simulink model "tigor_ev"  (R2020a)
settings: Solver=FixedStepDiscrete  StartTime=0.0  StopTime=0.4  RelTol=1e-3
InitFcn:
  | NAvg = 100;
  | Fs = 1e6;
  | FrameSize = 64;
libraries: dspsrcs4 x2, dspmisc x1
CloseFcn:
  | clear NAvg FrameSize Fs
settings Model: SnapshotInterval=1  Creator=The MathWorks, Inc.  LastModifiedBy=sateeshk
settings DataIOCC: LimitDataPoints=on  SaveFormat=Array  SaveOutput=off  SignalLogging=off  DSMLogging=off  SaveTime=off  ReturnWorkspaceOutputs=off
settings OptimizationCC: LifeSpan=inf
settings DebuggingCC: SolverPrmCheckMsg=warning  AllowSymbolicDim=off  SFUnexpectedBacktrackingDiag=warning  SFNoUnconditionalDefaultTransitionDiag=warning  SFExecutionAtInitializationDiag=none  ArithmeticOperatorsInVariantConditions=warning
settings HardwareCC: ProdBitPerPointer=32  ProdBitPerSizeT=32  ProdBitPerPtrDiffT=32  ProdLargestAtomicFloat=None  ProdIntDivRoundTo=Undefined  ProdEndianess=Unspecified  ProdWordSize=32  ProdHWDeviceType=32-bit Generic
settings ModelReferenceCC: PropagateSignalLabelsOutOfModel=off
settings SFSimCC: SimUseLocalCustomCode=off  CustomCodeUndefinedFunction=UseInterfaceOnly
settings RTWCC: RTWUseLocalCustomCode=off
settings CodeAppCC: StateflowObjectComments=on
settings GRTTargetCC: TargetLangStandard=C89/C90 (ANSI)
settings ConfigComp: CovMetricSettings=dw  CovHtmlReporting=on  CovSaveCumulativeToWorkspaceVar=on  CovSaveSingleToWorkspaceVar=on  CovExternalEMLEnable=off  CovSFcnEnable=off

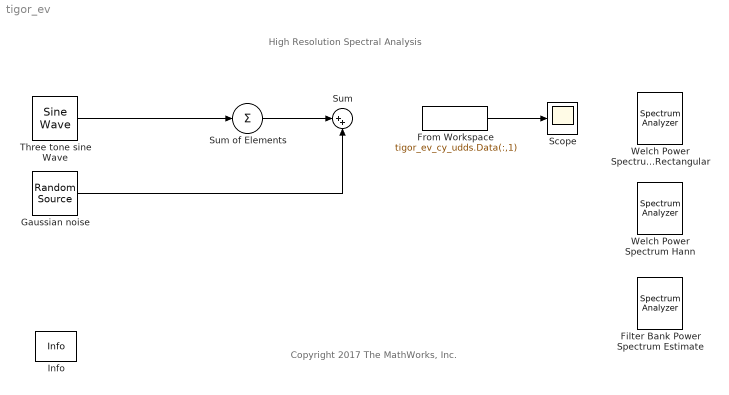
== system tigor_ev ==
  note: High Resolution Spectral Analysis
  note: Copyright 2017 The MathWorks, Inc.
  Filter Bank Power Spectrum Estimate : SpectrumAnalyzer
  From Workspace : FromWorkspace  VariableName=tigor_ev_cy_udds.Data(:,1)  SampleTime=-1
  Gaussian noise : dspsrcs4/Random Source  SrcType=Gaussian  NormMethod=Ziggurat  CltLength=12  MinVal=0  MaxVal=1  MeanVal=0  VarVal=1e-11  RepMode=Specify seed  rawSeed=1  IsInherit=off  SampMode=Discrete  SampTime=1/Fs  SampFrame=FrameSize  DataType=Double  OutComplex=Real  OutputFrames=off
  Info : dspmisc/Info  SystemSampleTime=-1  Latency=0  AutoFrameSizeCalculation=off
      settings: SourceProductBaseCode=DS
  Scope : Scope
  Sum : Sum  Inputs=|++
  Sum of Elements : Sum  Inputs=+  CollapseMode=Specified dimension  CollapseDim=2
  Three tone sine Wave : dspsrcs4/Sine Wave  Amplitude=[1e-5 1 2]  Frequency=[170000 200000 205000]  Phase=0  SampleMode=Discrete  OutComplex=Real  CompMethod=Trigonometric fcn  TableSize=Speed  SampleTime=1/Fs  SamplesPerFrame=FrameSize  ResetState=Restart at time zero  OutputFrames=off  dataType=double  wordLen=16  udDataType=sfix(16)  fracBitsMode=Best precision  numFracBits=15  OutDataTypeStr=double  LastOutDataTypeStr=double
  Welch Power Spectrum Hann : SpectrumAnalyzer
  Welch Power Spectrum Rectangular : SpectrumAnalyzer
  wires:
  Three tone sine Wave/1 -> Sum of Elements/1
  Sum of Elements/1 -> Sum/1
  Gaussian noise/1 -> Sum/2
  From Workspace/1 -> Scope/1
